simulink model "PowerStep01"  (R2015a)
settings: Solver=FixedStepDiscrete  SolverMode=SingleTasking  StartTime=0.0  StopTime=10.0  FixedStep=1e-3  RelTol=1e-3
libraries: simulink x1, mbed_spi_power x1, mbed_lib x1
settings Model: Creator=Stuv  LastModifiedBy=Stuv
settings OptimizationCC: OptimizeModelRefInitCode=on  LifeSpan=1
settings HardwareCC: ProdLargestAtomicInteger=Long  ProdLargestAtomicFloat=Double  ProdEndianess=LittleEndian  ProdHWDeviceType=ARM Compatible->ARM Cortex
settings RTWCC: SystemTargetFile=mbed.tlc  TemplateMakefile=mbed.tmf  Description=Mbed Target (Embedded Target)  TargetLang=C++
settings CodeAppCC: IgnoreCustomStorageClasses=off
settings STFCustomTargetCC: CombineOutputUpdateFcns=on  SupportContinuousTime=off  SupportVariableSizeSignals=off  SystemTargetFile=mbed.tlc
settings ERTTargetCC: SupportContinuousTime=off  SupportVariableSizeSignals=off  ERTCustomFileTemplate=mbed_file_process.tlc

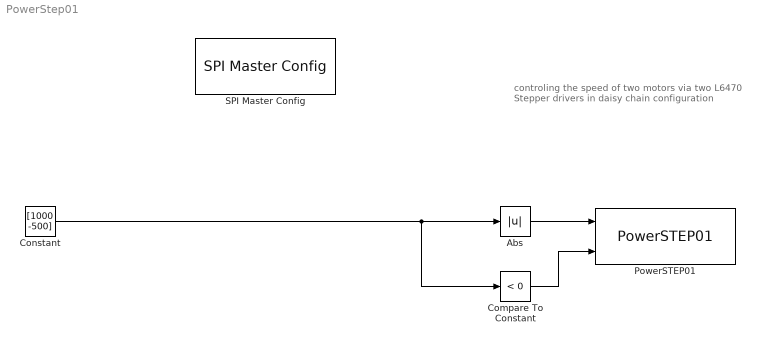
== system PowerStep01 ==
  note: controling the speed of two motors
      | via two L6470 Stepper drivers in
      | daisy chain configuration
  Abs : Abs
  Compare To Constant : simulink/Logic and Bit Operations/Compare To Constant  relop=<  const=0  OutDataTypeStr=uint8
  Constant : Constant  Value=[1000 -500]  OutDataTypeStr=single
  PowerSTEP01 : mbed_spi_power/PowerSTEP01  SpiPort=1  CsPort=A  CsPin=4  RstPort=B  RstPin=5  Cmd=Run  NumMotors=2  Acc=[100 100]  Dec=[100 100]  MaxSpd=[10000 10000]  MinSpd=[0 0]  StepMode_=1/64 Step  Voltage_real=[23 23]
  SPI Master Config : mbed_lib/SPI/SPI Master Config  Priority=0  SpiPort=1  SParameter6=100000  SParameter2=A  SParameter3=7  SParameter4=A  SParameter5=6  SCK_PORT=B  SCK_PIN=3
  wires:
  Constant/1 -> Abs/1, Compare To Constant/1
  Compare To Constant/1 -> PowerSTEP01/2
  Abs/1 -> PowerSTEP01/1
